simulink model "Simulink_Sim"  (R2020a)
settings: Solver=ode15s  StartTime=0.0  StopTime=tend  MaxStep=1e-2  RelTol=1e-2
undefined symbols (not defined in the file or in its folder): b_ocp, CellParam, Istring, m_ocp, N, n_t, Q_vector, SOC0_vector, SOC_PID1, SOC_PID2, SOC_PID3, SOC_PID4, SOC_PID5, SOC_PID6, Vbus_PID1, Vbus_PID2, Vbus_PID3, Vbus_PID4, Vbus_PID5, Vbus_PID6, Zload
settings Model: Creator=kawak  LastModifiedBy=kawak
settings SolverCC: ZeroCrossControl=DisableAll  SolverResetMethod=Robust

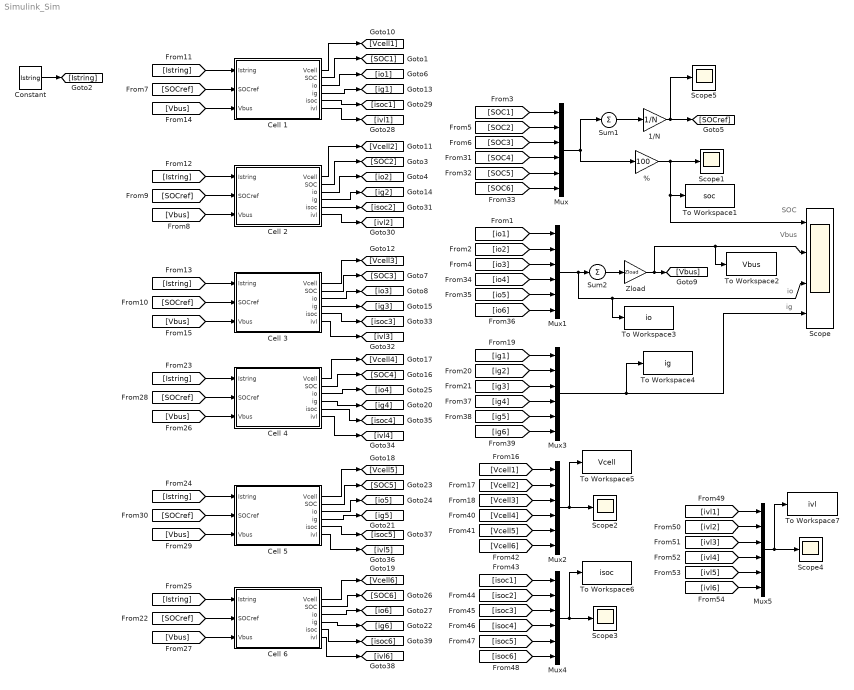
== system Simulink_Sim ==
  note: ig
  note: Vbus
  note: io
  note: SOC
  % : Gain  Gain=100
  1/N : Gain  Gain=1/N
  Cell 1 : Subsystem
  Cell 2 : Subsystem
  Cell 3 : Subsystem
  Cell 4 : Subsystem
  Cell 5 : Subsystem
  Cell 6 : Subsystem
  Constant : Constant  Value=Istring
  Mux{,1..5} (6 alike) : Mux  Inputs=6
  Scope : Scope  NumInputPorts=4
  Scope{1..5} (5 alike) : Scope
  Sum1 : Sum  Inputs=+
  Sum2 : Sum  Inputs=+
  To Workspace1 : ToWorkspace  VariableName=soc  SaveFormat=Structure With Time  SampleTime=-1
  To Workspace2 : ToWorkspace  VariableName=Vbus  SaveFormat=Structure With Time  SampleTime=-1
  To Workspace3 : ToWorkspace  VariableName=io  SaveFormat=Structure With Time  SampleTime=-1
  To Workspace4 : ToWorkspace  VariableName=ig  SaveFormat=Structure With Time  SampleTime=-1
  To Workspace5 : ToWorkspace  VariableName=Vcell  SaveFormat=Structure With Time  SampleTime=-1
  To Workspace6 : ToWorkspace  VariableName=isoc  SaveFormat=Structure With Time  SampleTime=-1
  To Workspace7 : ToWorkspace  VariableName=ivl  SaveFormat=Structure With Time  SampleTime=-1
  Zload : Gain  Gain=Zload
  wires:
  Sum1/1 -> 1/N/1
  Mux/1 -> Sum1/1, %/1
  [SOC1] -> Mux/1
  [SOC2] -> Mux/2
  [SOC3] -> Mux/3
  1/N/1 -> Scope5/1, [SOCref]
  Cell 1/2(SOC) -> [SOC1]
  Cell 1/3(io) -> [io1]
  Cell 3/3(io) -> [io3]
  Zload/1 -> To Workspace2/1, Scope/2, [Vbus]
  Mux1/1 -> To Workspace3/1, Scope/3, Sum2/1
  Sum2/1 -> Zload/1
  [Vbus] -> Cell 2/3(Vbus)
  [SOCref] -> Cell 1/2(SOCref)
  [SOCref] -> Cell 2/2(SOCref)
  [SOCref] -> Cell 3/2(SOCref)
  Constant/1 -> [Istring]
  [Istring] -> Cell 1/1(Istring)
  [Istring] -> Cell 2/1(Istring)
  [Istring] -> Cell 3/1(Istring)
  [Vbus] -> Cell 1/3(Vbus)
  [Vbus] -> Cell 3/3(Vbus)
  Cell 1/1(Vcell) -> [Vcell1]
  Cell 2/1(Vcell) -> [Vcell2]
  Cell 3/1(Vcell) -> [Vcell3]
  Cell 1/4(ig) -> [ig1]
  Cell 2/2(SOC) -> [SOC2]
  Cell 2/3(io) -> [io2]
  Cell 2/4(ig) -> [ig2]
  Cell 3/2(SOC) -> [SOC3]
  Cell 3/4(ig) -> [ig3]
  %/1 -> Scope1/1, To Workspace1/1, Scope/1
  Cell 6/3(io) -> [io6]
  [Istring] -> Cell 6/1(Istring)
  [SOCref] -> Cell 6/2(SOCref)
  Cell 6/2(SOC) -> [SOC6]
  Cell 6/1(Vcell) -> [Vcell6]
  Cell 5/4(ig) -> [ig5]
  Cell 5/2(SOC) -> [SOC5]
  Cell 5/1(Vcell) -> [Vcell5]
  [SOCref] -> Cell 5/2(SOCref)
  [Vbus] -> Cell 5/3(Vbus)
  [Istring] -> Cell 5/1(Istring)
  [Vbus] -> Cell 6/3(Vbus)
  Cell 4/4(ig) -> [ig4]
  Cell 4/3(io) -> [io4]
  [SOCref] -> Cell 4/2(SOCref)
  Cell 4/2(SOC) -> [SOC4]
  Cell 6/4(ig) -> [ig6]
  [Istring] -> Cell 4/1(Istring)
  Cell 4/1(Vcell) -> [Vcell4]
  [Vbus] -> Cell 4/3(Vbus)
  Cell 5/3(io) -> [io5]
  [SOC4] -> Mux/4
  [SOC5] -> Mux/5
  [SOC6] -> Mux/6
  [io1] -> Mux1/1
  [io2] -> Mux1/2
  [io3] -> Mux1/3
  [io4] -> Mux1/4
  [io5] -> Mux1/5
  [io6] -> Mux1/6
  [ig1] -> Mux3/1
  [ig2] -> Mux3/2
  [ig3] -> Mux3/3
  [ig4] -> Mux3/4
  [ig6] -> Mux3/6
  [ig5] -> Mux3/5
  Mux3/1 -> To Workspace4/1, Scope/4
  [Vcell1] -> Mux2/1
  [Vcell2] -> Mux2/2
  [Vcell3] -> Mux2/3
  [Vcell4] -> Mux2/4
  [Vcell5] -> Mux2/5
  [Vcell6] -> Mux2/6
  Mux2/1 -> To Workspace5/1, Scope2/1
  Cell 1/5(isoc) -> [isoc1]
  Cell 1/6(ivl) -> [ivl1]
  Cell 2/5(isoc) -> [isoc2]
  Cell 2/6(ivl) -> [ivl2]
  Cell 3/5(isoc) -> [isoc3]
  Cell 3/6(ivl) -> [ivl3]
  Cell 4/5(isoc) -> [isoc4]
  Cell 4/6(ivl) -> [ivl4]
  Cell 5/5(isoc) -> [isoc5]
  Cell 5/6(ivl) -> [ivl5]
  Cell 6/5(isoc) -> [isoc6]
  Cell 6/6(ivl) -> [ivl6]
  [isoc6] -> Mux4/6
  Mux4/1 -> To Workspace6/1, Scope3/1
  [isoc4] -> Mux4/4
  [isoc3] -> Mux4/3
  [isoc2] -> Mux4/2
  [isoc1] -> Mux4/1
  [isoc5] -> Mux4/5
  [ivl1] -> Mux5/1
  [ivl2] -> Mux5/2
  [ivl3] -> Mux5/3
  [ivl5] -> Mux5/5
  [ivl4] -> Mux5/4
  [ivl6] -> Mux5/6
  Mux5/1 -> To Workspace7/1, Scope4/1

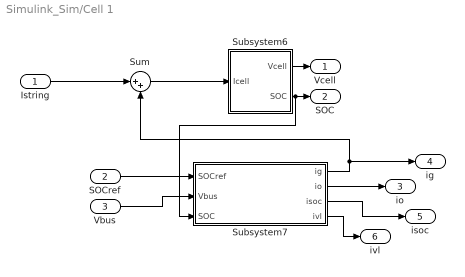
== system Simulink_Sim/Cell 1 ==
  Istring : Inport
  SOCref : Inport  Port=2
  Vbus : Inport  Port=3
  Subsystem6 : Subsystem  mask{SOC0=SOC0_vector(1), Q=Q_vector(1), R0=CellParam.R0, R1=CellParam.R1, RC=CellParam.RC, SOC=CellParam.tab_z, OCV=CellParam.tab_V}
      mask prompts: SOC0 "Initial SOC"; Q "Cell capacity"; SOC "SOC LUT"; OCV "OCV LUT"
  Subsystem7 : Subsystem  mask{m_ocp=m_ocp, b_ocp=b_ocp, n_t=n_t, SOC_PID=SOC_PID1, Vbus_PID=Vbus_PID1}
  Sum : Sum  Inputs=|++
  Vcell : Outport
  SOC : Outport  Port=2
  io : Outport  Port=3
  ig : Outport  Port=4
  isoc : Outport  Port=5
  ivl : Outport  Port=6
  wires:
  SOCref/1 -> Subsystem7/1(SOCref)
  Subsystem6/2(SOC) -> Subsystem7/3(SOC), SOC/1
  Subsystem6/1(Vcell) -> Vcell/1
  Vbus/1 -> Subsystem7/2(Vbus)
  Subsystem7/2(io) -> io/1
  Subsystem7/1(ig) -> ig/1, Sum/2
  Istring/1 -> Sum/1
  Sum/1 -> Subsystem6/1(Icell)
  Subsystem7/3(isoc) -> isoc/1
  Subsystem7/4(ivl) -> ivl/1

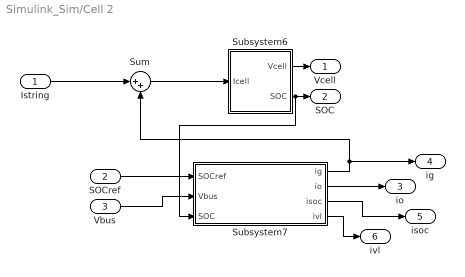
== system Simulink_Sim/Cell 2 ==
  Istring : Inport
  SOCref : Inport  Port=2
  Vbus : Inport  Port=3
  Subsystem6 : Subsystem  mask{SOC0=SOC0_vector(2), Q=Q_vector(2), R0=CellParam.R0, R1=CellParam.R1, RC=CellParam.RC, SOC=CellParam.tab_z, OCV=CellParam.tab_V}
      mask prompts: SOC0 "Initial SOC"; Q "Cell capacity"; SOC "SOC LUT"; OCV "OCV LUT"
  Subsystem7 : Subsystem  mask{m_ocp=m_ocp, b_ocp=b_ocp, n_t=n_t, SOC_PID=SOC_PID2, Vbus_PID=Vbus_PID2}
  Sum : Sum  Inputs=|++
  Vcell : Outport
  SOC : Outport  Port=2
  io : Outport  Port=3
  ig : Outport  Port=4
  isoc : Outport  Port=5
  ivl : Outport  Port=6
  wires:
  SOCref/1 -> Subsystem7/1(SOCref)
  Subsystem6/2(SOC) -> Subsystem7/3(SOC), SOC/1
  Subsystem6/1(Vcell) -> Vcell/1
  Vbus/1 -> Subsystem7/2(Vbus)
  Subsystem7/2(io) -> io/1
  Subsystem7/1(ig) -> ig/1, Sum/2
  Istring/1 -> Sum/1
  Sum/1 -> Subsystem6/1(Icell)
  Subsystem7/3(isoc) -> isoc/1
  Subsystem7/4(ivl) -> ivl/1

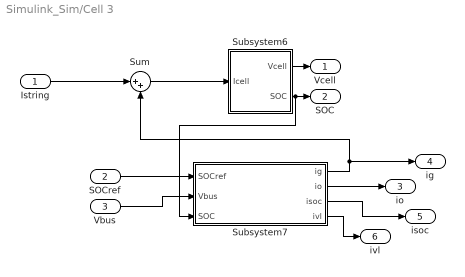
== system Simulink_Sim/Cell 3 ==
  Istring : Inport
  SOCref : Inport  Port=2
  Vbus : Inport  Port=3
  Subsystem6 : Subsystem  mask{SOC0=SOC0_vector(3), Q=Q_vector(3), R0=CellParam.R0, R1=CellParam.R1, RC=CellParam.RC, SOC=CellParam.tab_z, OCV=CellParam.tab_V}
      mask prompts: SOC0 "Initial SOC"; Q "Cell capacity"; SOC "SOC LUT"; OCV "OCV LUT"
  Subsystem7 : Subsystem  mask{m_ocp=m_ocp, b_ocp=b_ocp, n_t=n_t, SOC_PID=SOC_PID3, Vbus_PID=Vbus_PID3}
  Sum : Sum  Inputs=|++
  Vcell : Outport
  SOC : Outport  Port=2
  io : Outport  Port=3
  ig : Outport  Port=4
  isoc : Outport  Port=5
  ivl : Outport  Port=6
  wires:
  SOCref/1 -> Subsystem7/1(SOCref)
  Subsystem6/2(SOC) -> Subsystem7/3(SOC), SOC/1
  Subsystem6/1(Vcell) -> Vcell/1
  Vbus/1 -> Subsystem7/2(Vbus)
  Subsystem7/2(io) -> io/1
  Subsystem7/1(ig) -> ig/1, Sum/2
  Istring/1 -> Sum/1
  Sum/1 -> Subsystem6/1(Icell)
  Subsystem7/3(isoc) -> isoc/1
  Subsystem7/4(ivl) -> ivl/1

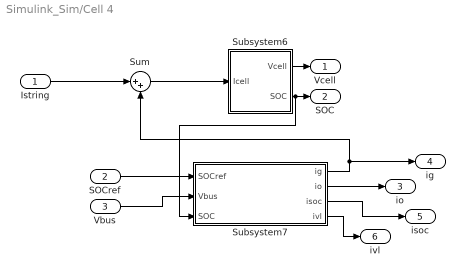
== system Simulink_Sim/Cell 4 ==
  Istring : Inport
  SOCref : Inport  Port=2
  Vbus : Inport  Port=3
  Subsystem6 : Subsystem  mask{SOC0=SOC0_vector(4), Q=Q_vector(4), R0=CellParam.R0, R1=CellParam.R1, RC=CellParam.RC, SOC=CellParam.tab_z, OCV=CellParam.tab_V}
      mask prompts: SOC0 "Initial SOC"; Q "Cell capacity"; SOC "SOC LUT"; OCV "OCV LUT"
  Subsystem7 : Subsystem  mask{m_ocp=m_ocp, b_ocp=b_ocp, n_t=n_t, SOC_PID=SOC_PID4, Vbus_PID=Vbus_PID4}
  Sum : Sum  Inputs=|++
  Vcell : Outport
  SOC : Outport  Port=2
  io : Outport  Port=3
  ig : Outport  Port=4
  isoc : Outport  Port=5
  ivl : Outport  Port=6
  wires:
  SOCref/1 -> Subsystem7/1(SOCref)
  Subsystem6/2(SOC) -> Subsystem7/3(SOC), SOC/1
  Subsystem6/1(Vcell) -> Vcell/1
  Vbus/1 -> Subsystem7/2(Vbus)
  Subsystem7/2(io) -> io/1
  Subsystem7/1(ig) -> ig/1, Sum/2
  Istring/1 -> Sum/1
  Sum/1 -> Subsystem6/1(Icell)
  Subsystem7/3(isoc) -> isoc/1
  Subsystem7/4(ivl) -> ivl/1

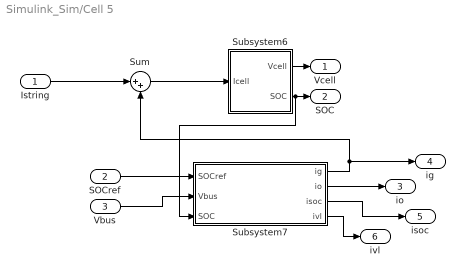
== system Simulink_Sim/Cell 5 ==
  Istring : Inport
  SOCref : Inport  Port=2
  Vbus : Inport  Port=3
  Subsystem6 : Subsystem  mask{SOC0=SOC0_vector(5), Q=Q_vector(5), R0=CellParam.R0, R1=CellParam.R1, RC=CellParam.RC, SOC=CellParam.tab_z, OCV=CellParam.tab_V}
      mask prompts: SOC0 "Initial SOC"; Q "Cell capacity"; SOC "SOC LUT"; OCV "OCV LUT"
  Subsystem7 : Subsystem  mask{m_ocp=m_ocp, b_ocp=b_ocp, n_t=n_t, SOC_PID=SOC_PID5, Vbus_PID=Vbus_PID5}
  Sum : Sum  Inputs=|++
  Vcell : Outport
  SOC : Outport  Port=2
  io : Outport  Port=3
  ig : Outport  Port=4
  isoc : Outport  Port=5
  ivl : Outport  Port=6
  wires:
  SOCref/1 -> Subsystem7/1(SOCref)
  Subsystem6/2(SOC) -> Subsystem7/3(SOC), SOC/1
  Subsystem6/1(Vcell) -> Vcell/1
  Vbus/1 -> Subsystem7/2(Vbus)
  Subsystem7/2(io) -> io/1
  Subsystem7/1(ig) -> ig/1, Sum/2
  Istring/1 -> Sum/1
  Sum/1 -> Subsystem6/1(Icell)
  Subsystem7/3(isoc) -> isoc/1
  Subsystem7/4(ivl) -> ivl/1

== system Simulink_Sim/Cell 6 ==
  Istring : Inport
  SOCref : Inport  Port=2
  Vbus : Inport  Port=3
  Subsystem6 : Subsystem  mask{SOC0=SOC0_vector(6), Q=Q_vector(6), R0=CellParam.R0, R1=CellParam.R1, RC=CellParam.RC, SOC=CellParam.tab_z, OCV=CellParam.tab_V}
      mask prompts: SOC0 "Initial SOC"; Q "Cell capacity"; SOC "SOC LUT"; OCV "OCV LUT"
  Subsystem7 : Subsystem  mask{m_ocp=m_ocp, b_ocp=b_ocp, n_t=n_t, SOC_PID=SOC_PID6, Vbus_PID=Vbus_PID6}
  Sum : Sum  Inputs=|++
  Vcell : Outport
  SOC : Outport  Port=2
  io : Outport  Port=3
  ig : Outport  Port=4
  isoc : Outport  Port=5
  ivl : Outport  Port=6
  wires:
  SOCref/1 -> Subsystem7/1(SOCref)
  Subsystem6/2(SOC) -> Subsystem7/3(SOC), SOC/1
  Subsystem6/1(Vcell) -> Vcell/1
  Vbus/1 -> Subsystem7/2(Vbus)
  Subsystem7/2(io) -> io/1
  Subsystem7/1(ig) -> ig/1, Sum/2
  Istring/1 -> Sum/1
  Sum/1 -> Subsystem6/1(Icell)
  Subsystem7/3(isoc) -> isoc/1
  Subsystem7/4(ivl) -> ivl/1

== system Simulink_Sim/Cell 1/Subsystem6 ==
  Icell : Inport
  1-D Lookup Table : Lookup_n-D  NumberOfTableDimensions=1  BreakpointsForDimension1=SOC  Table=OCV  InternalRulePriority=Speed  RndMeth=Simplest  InputSameDT=on
  Add : Sum  Inputs=+++
  Gain : Gain  Gain=1/(Q)
  Gain1 : Gain  Gain=R0
  Integrator : Integrator  InitialCondition=SOC0
  Transfer Fcn : TransferFcn  Numerator=[R1]  Denominator=[RC 1]
  Vcell : Outport
  SOC : Outport  Port=2
  wires:
  Gain1/1 -> Add/2
  Icell/1 -> Gain1/1, Transfer Fcn/1, Gain/1
  1-D Lookup Table/1 -> Add/1
  Integrator/1 -> SOC/1, 1-D Lookup Table/1
  Gain/1 -> Integrator/1
  Add/1 -> Vcell/1
  Transfer Fcn/1 -> Add/3

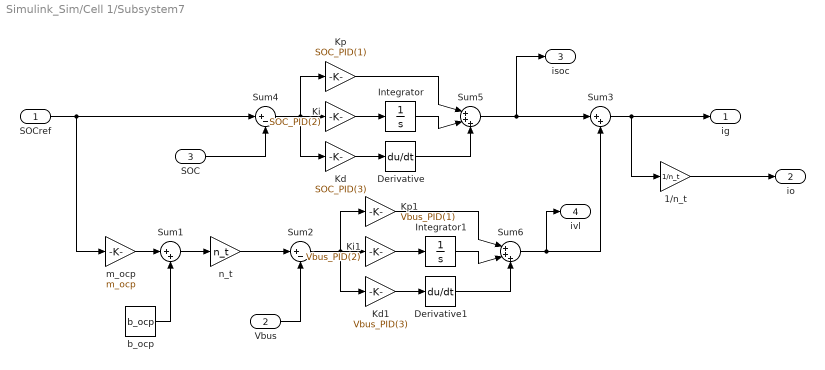
== system Simulink_Sim/Cell 1/Subsystem7 ==
  SOCref : Inport
  Vbus : Inport  Port=2
  SOC : Inport  Port=3
  1/n_t : Gain  Gain=1/n_t
  Derivative : Derivative
  Derivative1 : Derivative
  Integrator : Integrator
  Integrator1 : Integrator
  Kd : Gain  Gain=SOC_PID(3)
  Kd1 : Gain  Gain=Vbus_PID(3)
  Ki : Gain  Gain=SOC_PID(2)
  Ki1 : Gain  Gain=Vbus_PID(2)
  Kp : Gain  Gain=SOC_PID(1)
  Kp1 : Gain  Gain=Vbus_PID(1)
  Sum1 : Sum  Inputs=|++
  Sum2 : Sum  Inputs=|+-
  Sum3 : Sum  Inputs=|++
  Sum4 : Sum  Inputs=|+-
  Sum5 : Sum  Inputs=|+++
  Sum6 : Sum  Inputs=|+++
  b_ocp : Constant  Value=b_ocp
  m_ocp : Gain  Gain=m_ocp
  n_t : Gain  Gain=n_t
  ig : Outport
  io : Outport  Port=2
  isoc : Outport  Port=3
  ivl : Outport  Port=4
  wires:
  SOCref/1 -> Sum4/1, m_ocp/1
  n_t/1 -> Sum2/1
  b_ocp/1 -> Sum1/2
  Vbus/1 -> Sum2/2
  Sum3/1 -> ig/1, 1/n_t/1
  1/n_t/1 -> io/1
  Sum5/1 -> isoc/1, Sum3/1
  m_ocp/1 -> Sum1/1
  Sum1/1 -> n_t/1
  SOC/1 -> Sum4/2
  Sum4/1 -> Kd/1, Kp/1, Ki/1
  Kd/1 -> Derivative/1
  Ki/1 -> Integrator/1
  Kp/1 -> Sum5/1
  Integrator/1 -> Sum5/2
  Derivative/1 -> Sum5/3
  Sum2/1 -> Kd1/1, Kp1/1, Ki1/1
  Ki1/1 -> Integrator1/1
  Kd1/1 -> Derivative1/1
  Integrator1/1 -> Sum6/2
  Kp1/1 -> Sum6/1
  Derivative1/1 -> Sum6/3
  Sum6/1 -> ivl/1, Sum3/2

== system Simulink_Sim/Cell 2/Subsystem6 ==
  Icell : Inport
  1-D Lookup Table : Lookup_n-D  NumberOfTableDimensions=1  BreakpointsForDimension1=SOC  Table=OCV  InternalRulePriority=Speed  RndMeth=Simplest  InputSameDT=on
  Add : Sum  Inputs=+++
  Gain : Gain  Gain=1/(Q)
  Gain1 : Gain  Gain=R0
  Integrator : Integrator  InitialCondition=SOC0
  Transfer Fcn : TransferFcn  Numerator=[R1]  Denominator=[RC 1]
  Vcell : Outport
  SOC : Outport  Port=2
  wires:
  Gain1/1 -> Add/2
  Icell/1 -> Gain1/1, Transfer Fcn/1, Gain/1
  1-D Lookup Table/1 -> Add/1
  Integrator/1 -> SOC/1, 1-D Lookup Table/1
  Gain/1 -> Integrator/1
  Add/1 -> Vcell/1
  Transfer Fcn/1 -> Add/3

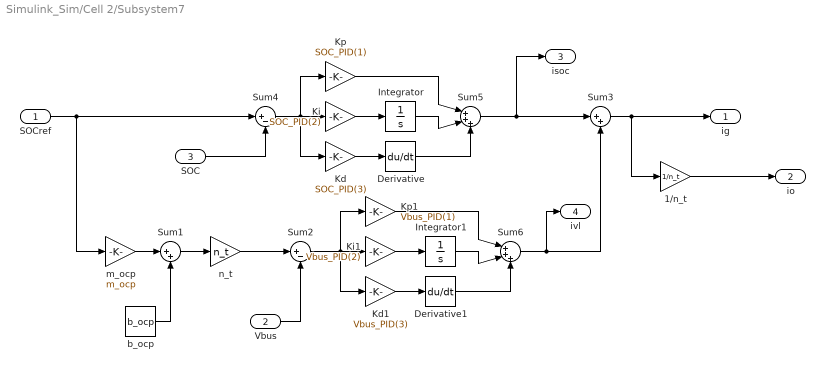
== system Simulink_Sim/Cell 2/Subsystem7 ==
  SOCref : Inport
  Vbus : Inport  Port=2
  SOC : Inport  Port=3
  1/n_t : Gain  Gain=1/n_t
  Derivative : Derivative
  Derivative1 : Derivative
  Integrator : Integrator
  Integrator1 : Integrator
  Kd : Gain  Gain=SOC_PID(3)
  Kd1 : Gain  Gain=Vbus_PID(3)
  Ki : Gain  Gain=SOC_PID(2)
  Ki1 : Gain  Gain=Vbus_PID(2)
  Kp : Gain  Gain=SOC_PID(1)
  Kp1 : Gain  Gain=Vbus_PID(1)
  Sum1 : Sum  Inputs=|++
  Sum2 : Sum  Inputs=|+-
  Sum3 : Sum  Inputs=|++
  Sum4 : Sum  Inputs=|+-
  Sum5 : Sum  Inputs=|+++
  Sum6 : Sum  Inputs=|+++
  b_ocp : Constant  Value=b_ocp
  m_ocp : Gain  Gain=m_ocp
  n_t : Gain  Gain=n_t
  ig : Outport
  io : Outport  Port=2
  isoc : Outport  Port=3
  ivl : Outport  Port=4
  wires:
  SOCref/1 -> Sum4/1, m_ocp/1
  n_t/1 -> Sum2/1
  b_ocp/1 -> Sum1/2
  Vbus/1 -> Sum2/2
  Sum3/1 -> ig/1, 1/n_t/1
  1/n_t/1 -> io/1
  Sum5/1 -> isoc/1, Sum3/1
  m_ocp/1 -> Sum1/1
  Sum1/1 -> n_t/1
  SOC/1 -> Sum4/2
  Sum4/1 -> Kd/1, Kp/1, Ki/1
  Kd/1 -> Derivative/1
  Ki/1 -> Integrator/1
  Kp/1 -> Sum5/1
  Integrator/1 -> Sum5/2
  Derivative/1 -> Sum5/3
  Sum2/1 -> Kd1/1, Kp1/1, Ki1/1
  Ki1/1 -> Integrator1/1
  Kd1/1 -> Derivative1/1
  Integrator1/1 -> Sum6/2
  Kp1/1 -> Sum6/1
  Derivative1/1 -> Sum6/3
  Sum6/1 -> ivl/1, Sum3/2

== system Simulink_Sim/Cell 3/Subsystem6 ==
  Icell : Inport
  1-D Lookup Table : Lookup_n-D  NumberOfTableDimensions=1  BreakpointsForDimension1=SOC  Table=OCV  InternalRulePriority=Speed  RndMeth=Simplest  InputSameDT=on
  Add : Sum  Inputs=+++
  Gain : Gain  Gain=1/(Q)
  Gain1 : Gain  Gain=R0
  Integrator : Integrator  InitialCondition=SOC0
  Transfer Fcn : TransferFcn  Numerator=[R1]  Denominator=[RC 1]
  Vcell : Outport
  SOC : Outport  Port=2
  wires:
  Gain1/1 -> Add/2
  Icell/1 -> Gain1/1, Transfer Fcn/1, Gain/1
  1-D Lookup Table/1 -> Add/1
  Integrator/1 -> SOC/1, 1-D Lookup Table/1
  Gain/1 -> Integrator/1
  Add/1 -> Vcell/1
  Transfer Fcn/1 -> Add/3

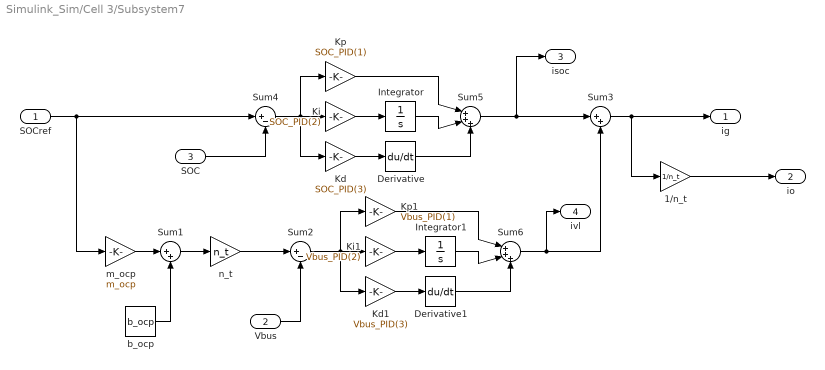
== system Simulink_Sim/Cell 3/Subsystem7 ==
  SOCref : Inport
  Vbus : Inport  Port=2
  SOC : Inport  Port=3
  1/n_t : Gain  Gain=1/n_t
  Derivative : Derivative
  Derivative1 : Derivative
  Integrator : Integrator
  Integrator1 : Integrator
  Kd : Gain  Gain=SOC_PID(3)
  Kd1 : Gain  Gain=Vbus_PID(3)
  Ki : Gain  Gain=SOC_PID(2)
  Ki1 : Gain  Gain=Vbus_PID(2)
  Kp : Gain  Gain=SOC_PID(1)
  Kp1 : Gain  Gain=Vbus_PID(1)
  Sum1 : Sum  Inputs=|++
  Sum2 : Sum  Inputs=|+-
  Sum3 : Sum  Inputs=|++
  Sum4 : Sum  Inputs=|+-
  Sum5 : Sum  Inputs=|+++
  Sum6 : Sum  Inputs=|+++
  b_ocp : Constant  Value=b_ocp
  m_ocp : Gain  Gain=m_ocp
  n_t : Gain  Gain=n_t
  ig : Outport
  io : Outport  Port=2
  isoc : Outport  Port=3
  ivl : Outport  Port=4
  wires:
  SOCref/1 -> Sum4/1, m_ocp/1
  n_t/1 -> Sum2/1
  b_ocp/1 -> Sum1/2
  Vbus/1 -> Sum2/2
  Sum3/1 -> ig/1, 1/n_t/1
  1/n_t/1 -> io/1
  Sum5/1 -> isoc/1, Sum3/1
  m_ocp/1 -> Sum1/1
  Sum1/1 -> n_t/1
  SOC/1 -> Sum4/2
  Sum4/1 -> Kd/1, Kp/1, Ki/1
  Kd/1 -> Derivative/1
  Ki/1 -> Integrator/1
  Kp/1 -> Sum5/1
  Integrator/1 -> Sum5/2
  Derivative/1 -> Sum5/3
  Sum2/1 -> Kd1/1, Kp1/1, Ki1/1
  Ki1/1 -> Integrator1/1
  Kd1/1 -> Derivative1/1
  Integrator1/1 -> Sum6/2
  Kp1/1 -> Sum6/1
  Derivative1/1 -> Sum6/3
  Sum6/1 -> ivl/1, Sum3/2

== system Simulink_Sim/Cell 4/Subsystem6 ==
  Icell : Inport
  1-D Lookup Table : Lookup_n-D  NumberOfTableDimensions=1  BreakpointsForDimension1=SOC  Table=OCV  InternalRulePriority=Speed  RndMeth=Simplest  InputSameDT=on
  Add : Sum  Inputs=+++
  Gain : Gain  Gain=1/(Q)
  Gain1 : Gain  Gain=R0
  Integrator : Integrator  InitialCondition=SOC0
  Transfer Fcn : TransferFcn  Numerator=[R1]  Denominator=[RC 1]
  Vcell : Outport
  SOC : Outport  Port=2
  wires:
  Gain1/1 -> Add/2
  Icell/1 -> Gain1/1, Transfer Fcn/1, Gain/1
  1-D Lookup Table/1 -> Add/1
  Integrator/1 -> SOC/1, 1-D Lookup Table/1
  Gain/1 -> Integrator/1
  Add/1 -> Vcell/1
  Transfer Fcn/1 -> Add/3

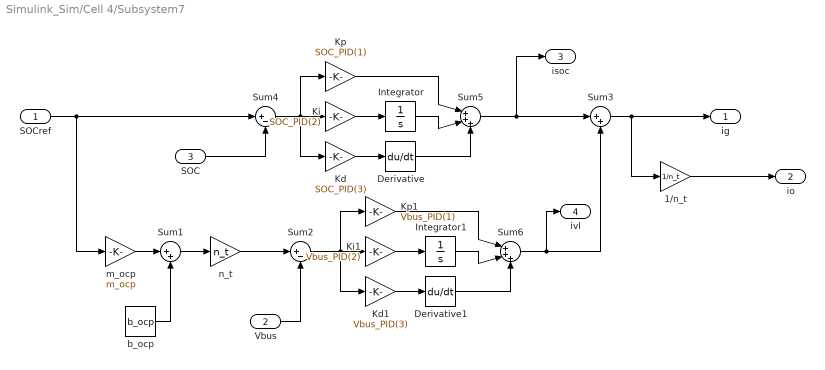
== system Simulink_Sim/Cell 4/Subsystem7 ==
  SOCref : Inport
  Vbus : Inport  Port=2
  SOC : Inport  Port=3
  1/n_t : Gain  Gain=1/n_t
  Derivative : Derivative
  Derivative1 : Derivative
  Integrator : Integrator
  Integrator1 : Integrator
  Kd : Gain  Gain=SOC_PID(3)
  Kd1 : Gain  Gain=Vbus_PID(3)
  Ki : Gain  Gain=SOC_PID(2)
  Ki1 : Gain  Gain=Vbus_PID(2)
  Kp : Gain  Gain=SOC_PID(1)
  Kp1 : Gain  Gain=Vbus_PID(1)
  Sum1 : Sum  Inputs=|++
  Sum2 : Sum  Inputs=|+-
  Sum3 : Sum  Inputs=|++
  Sum4 : Sum  Inputs=|+-
  Sum5 : Sum  Inputs=|+++
  Sum6 : Sum  Inputs=|+++
  b_ocp : Constant  Value=b_ocp
  m_ocp : Gain  Gain=m_ocp
  n_t : Gain  Gain=n_t
  ig : Outport
  io : Outport  Port=2
  isoc : Outport  Port=3
  ivl : Outport  Port=4
  wires:
  SOCref/1 -> Sum4/1, m_ocp/1
  n_t/1 -> Sum2/1
  b_ocp/1 -> Sum1/2
  Vbus/1 -> Sum2/2
  Sum3/1 -> ig/1, 1/n_t/1
  1/n_t/1 -> io/1
  Sum5/1 -> isoc/1, Sum3/1
  m_ocp/1 -> Sum1/1
  Sum1/1 -> n_t/1
  SOC/1 -> Sum4/2
  Sum4/1 -> Kd/1, Kp/1, Ki/1
  Kd/1 -> Derivative/1
  Ki/1 -> Integrator/1
  Kp/1 -> Sum5/1
  Integrator/1 -> Sum5/2
  Derivative/1 -> Sum5/3
  Sum2/1 -> Kd1/1, Kp1/1, Ki1/1
  Ki1/1 -> Integrator1/1
  Kd1/1 -> Derivative1/1
  Integrator1/1 -> Sum6/2
  Kp1/1 -> Sum6/1
  Derivative1/1 -> Sum6/3
  Sum6/1 -> ivl/1, Sum3/2

== system Simulink_Sim/Cell 5/Subsystem6 ==
  Icell : Inport
  1-D Lookup Table : Lookup_n-D  NumberOfTableDimensions=1  BreakpointsForDimension1=SOC  Table=OCV  InternalRulePriority=Speed  RndMeth=Simplest  InputSameDT=on
  Add : Sum  Inputs=+++
  Gain : Gain  Gain=1/(Q)
  Gain1 : Gain  Gain=R0
  Integrator : Integrator  InitialCondition=SOC0
  Transfer Fcn : TransferFcn  Numerator=[R1]  Denominator=[RC 1]
  Vcell : Outport
  SOC : Outport  Port=2
  wires:
  Gain1/1 -> Add/2
  Icell/1 -> Gain1/1, Transfer Fcn/1, Gain/1
  1-D Lookup Table/1 -> Add/1
  Integrator/1 -> SOC/1, 1-D Lookup Table/1
  Gain/1 -> Integrator/1
  Add/1 -> Vcell/1
  Transfer Fcn/1 -> Add/3

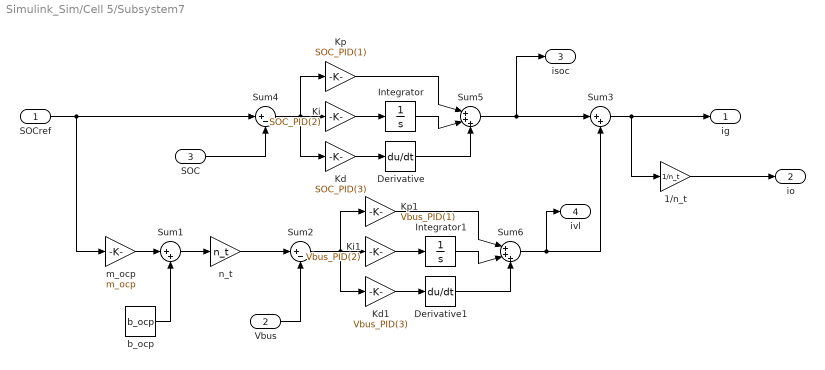
== system Simulink_Sim/Cell 5/Subsystem7 ==
  SOCref : Inport
  Vbus : Inport  Port=2
  SOC : Inport  Port=3
  1/n_t : Gain  Gain=1/n_t
  Derivative : Derivative
  Derivative1 : Derivative
  Integrator : Integrator
  Integrator1 : Integrator
  Kd : Gain  Gain=SOC_PID(3)
  Kd1 : Gain  Gain=Vbus_PID(3)
  Ki : Gain  Gain=SOC_PID(2)
  Ki1 : Gain  Gain=Vbus_PID(2)
  Kp : Gain  Gain=SOC_PID(1)
  Kp1 : Gain  Gain=Vbus_PID(1)
  Sum1 : Sum  Inputs=|++
  Sum2 : Sum  Inputs=|+-
  Sum3 : Sum  Inputs=|++
  Sum4 : Sum  Inputs=|+-
  Sum5 : Sum  Inputs=|+++
  Sum6 : Sum  Inputs=|+++
  b_ocp : Constant  Value=b_ocp
  m_ocp : Gain  Gain=m_ocp
  n_t : Gain  Gain=n_t
  ig : Outport
  io : Outport  Port=2
  isoc : Outport  Port=3
  ivl : Outport  Port=4
  wires:
  SOCref/1 -> Sum4/1, m_ocp/1
  n_t/1 -> Sum2/1
  b_ocp/1 -> Sum1/2
  Vbus/1 -> Sum2/2
  Sum3/1 -> ig/1, 1/n_t/1
  1/n_t/1 -> io/1
  Sum5/1 -> isoc/1, Sum3/1
  m_ocp/1 -> Sum1/1
  Sum1/1 -> n_t/1
  SOC/1 -> Sum4/2
  Sum4/1 -> Kd/1, Kp/1, Ki/1
  Kd/1 -> Derivative/1
  Ki/1 -> Integrator/1
  Kp/1 -> Sum5/1
  Integrator/1 -> Sum5/2
  Derivative/1 -> Sum5/3
  Sum2/1 -> Kd1/1, Kp1/1, Ki1/1
  Ki1/1 -> Integrator1/1
  Kd1/1 -> Derivative1/1
  Integrator1/1 -> Sum6/2
  Kp1/1 -> Sum6/1
  Derivative1/1 -> Sum6/3
  Sum6/1 -> ivl/1, Sum3/2

== system Simulink_Sim/Cell 6/Subsystem6 ==
  Icell : Inport
  1-D Lookup Table : Lookup_n-D  NumberOfTableDimensions=1  BreakpointsForDimension1=SOC  Table=OCV  InternalRulePriority=Speed  RndMeth=Simplest  InputSameDT=on
  Add : Sum  Inputs=+++
  Gain : Gain  Gain=1/(Q)
  Gain1 : Gain  Gain=R0
  Integrator : Integrator  InitialCondition=SOC0
  Transfer Fcn : TransferFcn  Numerator=[R1]  Denominator=[RC 1]
  Vcell : Outport
  SOC : Outport  Port=2
  wires:
  Gain1/1 -> Add/2
  Icell/1 -> Gain1/1, Transfer Fcn/1, Gain/1
  1-D Lookup Table/1 -> Add/1
  Integrator/1 -> SOC/1, 1-D Lookup Table/1
  Gain/1 -> Integrator/1
  Add/1 -> Vcell/1
  Transfer Fcn/1 -> Add/3

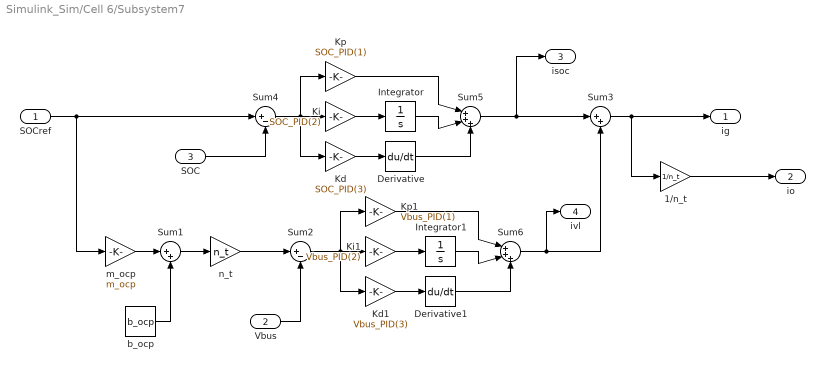
== system Simulink_Sim/Cell 6/Subsystem7 ==
  SOCref : Inport
  Vbus : Inport  Port=2
  SOC : Inport  Port=3
  1/n_t : Gain  Gain=1/n_t
  Derivative : Derivative
  Derivative1 : Derivative
  Integrator : Integrator
  Integrator1 : Integrator
  Kd : Gain  Gain=SOC_PID(3)
  Kd1 : Gain  Gain=Vbus_PID(3)
  Ki : Gain  Gain=SOC_PID(2)
  Ki1 : Gain  Gain=Vbus_PID(2)
  Kp : Gain  Gain=SOC_PID(1)
  Kp1 : Gain  Gain=Vbus_PID(1)
  Sum1 : Sum  Inputs=|++
  Sum2 : Sum  Inputs=|+-
  Sum3 : Sum  Inputs=|++
  Sum4 : Sum  Inputs=|+-
  Sum5 : Sum  Inputs=|+++
  Sum6 : Sum  Inputs=|+++
  b_ocp : Constant  Value=b_ocp
  m_ocp : Gain  Gain=m_ocp
  n_t : Gain  Gain=n_t
  ig : Outport
  io : Outport  Port=2
  isoc : Outport  Port=3
  ivl : Outport  Port=4
  wires:
  SOCref/1 -> Sum4/1, m_ocp/1
  n_t/1 -> Sum2/1
  b_ocp/1 -> Sum1/2
  Vbus/1 -> Sum2/2
  Sum3/1 -> ig/1, 1/n_t/1
  1/n_t/1 -> io/1
  Sum5/1 -> isoc/1, Sum3/1
  m_ocp/1 -> Sum1/1
  Sum1/1 -> n_t/1
  SOC/1 -> Sum4/2
  Sum4/1 -> Kd/1, Kp/1, Ki/1
  Kd/1 -> Derivative/1
  Ki/1 -> Integrator/1
  Kp/1 -> Sum5/1
  Integrator/1 -> Sum5/2
  Derivative/1 -> Sum5/3
  Sum2/1 -> Kd1/1, Kp1/1, Ki1/1
  Ki1/1 -> Integrator1/1
  Kd1/1 -> Derivative1/1
  Integrator1/1 -> Sum6/2
  Kp1/1 -> Sum6/1
  Derivative1/1 -> Sum6/3
  Sum6/1 -> ivl/1, Sum3/2
